simulink model "CBE_145_HW4_P1a"  (R2021b)
settings: Solver=VariableStepAuto  StartTime=0.0  StopTime=25  RelTol=1e-3
settings Model: Creator=Jesus Vergara  LastModifiedBy=brame
settings SolverCC: AlgebraicLoopSolver=TrustRegion
settings DebuggingCC: SFMachineParentedDataDiag=warning

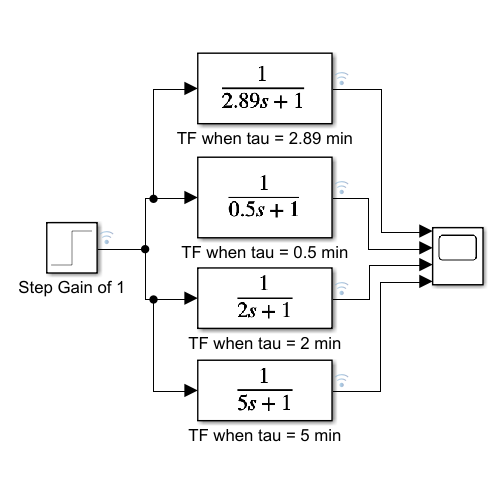
[thumbnail: Simulink's stored preview of the top-level diagram]
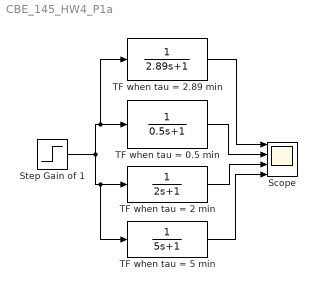
== system CBE_145_HW4_P1a ==
  Scope : Scope  NumInputPorts=4
  Step Gain of 1 : Step  SampleTime=0
  TF when tau = 0.5 min : TransferFcn  Denominator=[0.5 1]
  TF when tau = 2 min : TransferFcn  Denominator=[2 1]
  TF when tau = 2.89 min : TransferFcn  Denominator=[2.89 1]
  TF when tau = 5 min : TransferFcn  Denominator=[5 1]
  wires:
  TF when tau = 2.89 min/1 -> Scope/1
  TF when tau = 0.5 min/1 -> Scope/2
  TF when tau = 2 min/1 -> Scope/3
  TF when tau = 5 min/1 -> Scope/4
  Step Gain of 1/1 -> TF when tau = 2.89 min/1, TF when tau = 0.5 min/1, TF when tau = 5 min/1, TF when tau = 2 min/1
